simulink library "mech_car_library"  (Simulink 7.1)
libraries: mblibv1 x13, mwlibrary x10, simulink x5
settings Model: Creator=dsampson  LastModifiedBy=batserve

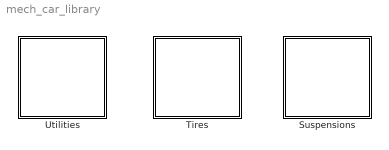
== system mech_car_library ==
  Suspensions : Subsystem
  Tires : Subsystem
  Utilities : Subsystem

== system mech_car_library/Suspensions ==
  Suspension 1 : Subsystem  Orientation=left  mask{r=0.742, d=2, h_u=0.53, k=190e3, b=2025, m_u=706, I_xx_u=0, I_yy_u=440}
      mask prompts: r "Roll centre height [m]:"; d "Track width [m]:"; h_u "Wheel radius [m]:"; k "Suspension stiffness [N/m]:"; b "Suspension damping [N.s/m]:"; m_u "Mass [kg]:"; I_xx_u "Roll inertia [kg.m2]:"; I_yy_u "Yaw inertia [kg.m2]:"
      mask init:
      | I_zz_u = I_xx_u;

== system mech_car_library/Tires ==
  Magic 1 : Subsystem  mask{r_e=0.53, r_f=0.55, m_w=10, F_z=25000, F_x_max=15000, kappa_max=10, F_y_max=15000, alpha_max=10, sigma_k=1.6, kt=1030000}
      mask prompts: r_e "Effective rolling radius [m]:"; r_f "Unloaded radius [m]:"; m_w "Wheel mass [kg]:"; F_z "Rated vertical load [N]:"; F_x_max "Peak longitudinal force at rated load [N]:"; kappa_max "Best slip at rated load [percent]:"; F_y_max "Peak lateral force at rated load [N]:"; alpha_max "Best sideslip at rated load [deg]:"; sigma_k "Relaxation length at rated load [m]:"; kt "Vertical stiffness"

== system mech_car_library/Utilities ==
  Cross Product : Subsystem
      mask Type: Cross Product
      mask Description: Calculate the cross product of two 3x1 vectors.
  Unit Vector : Subsystem
      mask Type: Unit Vector
      mask Description: Normalize a 3x1 vector.

== system mech_car_library/Suspensions/Suspension 1 ==
  Body Spring & Damper : mblibv1/Force  Elements/Body Spring & Damper  Orientation=down  DialogController=MECH.DynMechDlgSource  SystemSampleTime=-1  DialogClass=BodySpringDamper  Spring_k=k  Damper_b=b  Offset_x0=0  PositionUnits=m  VelocityUnits=m/s  ForceUnits=N
  Body Spring & Damper1 : mblibv1/Force  Elements/Body Spring & Damper  Orientation=down  DialogController=MECH.DynMechDlgSource  SystemSampleTime=-1  DialogClass=BodySpringDamper  Spring_k=k  Damper_b=b  Offset_x0=0  PositionUnits=m  VelocityUnits=m/s  ForceUnits=N
  Body1 : mblibv1/Bodies/Body  Orientation=down  DialogController=MECH.DynMechDlgSource  PhysicalDomain=mechanical  SubClassName=Unknown  LeftPortType=workingframe  RightPortType=workingframe  LConnTagsString=CS1|CS2|CS3  RConnTagsString=CS4|CS5  DialogClass=MechanicalBodyBlock  Mass=m_u  MassUnits=kg  InertiaUnits=kg*m^2  Inertia=diag([I_xx_u,I_yy_u,I_zz_u])  Shape=Cylinder  ShapeDims=[1 1]  ShapeUnits=m  ShapeUse=false  Density=1  DensityUnits=kg/m^3  DensityUse=false  GraphicsMode=1  BodyColor=[0.5 0.5 0.5]  GraphicsObj=[]  AttachedToCS=1  CG=Left$CG$[0 0 0]$CS2$CS2$m$[0 0 0]$Euler X-Y-Z$deg$WORLD$false  WorkingFrames=Left$CS1$[0,d/2,0]$CS2$CS2$m$[0 0 0]$Euler X-Y-Z$deg$WORLD$true#Left$CS2$[0,0,0]$ADJOINING$ADJOINING$m$[0 0 0]$Euler X-Y-Z$deg$WORLD$true#Left$CS3$[0,-d/2,0]$CS2$CS2$m$[0 0 0]$Euler X-Y-Z$deg$WORLD$true#Right$CS4$[0,d/2,h_u-r]$CS2$CS2$m$[0 0 0]$Euler X-Y-Z$deg$WORLD$true#Right$CS5$[0,-d/2,h_u-r]$CS2$CS2$m$[0 0 0]$Euler X-Y-Z$deg$WORLD$true  CGPos=[0 0 0]  CGRot=[0 0 0]  CS0Pos=[]  CS0Rot=[]  CS1Pos=[0 0 0]  CS1Rot=[0 0 0]  CS2Pos=[0 0 0]  CS2Rot=[0 0 0]  CS3Pos=[]  CS3Rot=[]  CS4Pos=[]  CS4Rot=[]  CS5Pos=[]  CS5Rot=[]  CS6Pos=[]  CS6Rot=[]  CS7Pos=[]  CS7Rot=[]  CS8Pos=[]  CS8Rot=[]  CS9Pos=[]  CS9Rot=[]  CS10Pos=[]  CS10Rot=[]  CS11Pos=[]  CS11Rot=[]  CS12Pos=[]  CS12Rot=[]  CS13Pos=[]  CS13Rot=[]  CS14Pos=[]  CS14Rot=[]  CS15Pos=[]  CS15Rot=[]  CS16Pos=[]  CS16Rot=[]  CS17Pos=[]  CS17Rot=[]  CS18Pos=[]  CS18Rot=[]  CS19Pos=[]  CS19Rot=[]  CS20Pos=[]  CS20Rot=[]
  Custom Joint : mblibv1/Joints/Custom Joint  Orientation=down  DialogController=MECH.DynMechDlgSource  PhysicalDomain=mechanical  SubClassName=custom_joint  LeftPortType=blob  RightPortType=blob  LConnTagsString=__newl0  RConnTagsString=__newr0  NumSAPorts=0  CutJoint=off  MarkAsCut=off  Primitives=prismatic_revolute  PrimitiveProps=P1$Base$[0 0 1]$prismatic#R1$Base$[1 0 0]$revolute  DialogClass=JointBlock  R1Axis=[1 0 0]  R2Axis=[]  R3Axis=[]  P1Axis=[]  P2Axis=[]  P3Axis=[]  SAxis=[]
  Left Spring : PMIOPort  Orientation=down  Port=1  Side=Left
  Joint : PMIOPort  Orientation=down  Port=2  Side=Left
  Right Spring : PMIOPort  Orientation=down  Port=3  Side=Left
  Left Wheel : PMIOPort  Orientation=up  Port=4  Side=Right
  Right Wheel : PMIOPort  Orientation=up  Port=5  Side=Right
  connections:
  Body Spring & Damper/RConn1 -- Body1/LConn1
  Body Spring & Damper1/RConn1 -- Body1/LConn3
  Custom Joint/RConn1 -- Body1/LConn2
  Left Spring/RConn1 -- Body Spring & Damper/LConn1
  Right Spring/RConn1 -- Body Spring & Damper1/LConn1
  Joint/RConn1 -- Custom Joint/LConn1
  Left Wheel/RConn1 -- Body1/RConn1
  Right Wheel/RConn1 -- Body1/RConn2

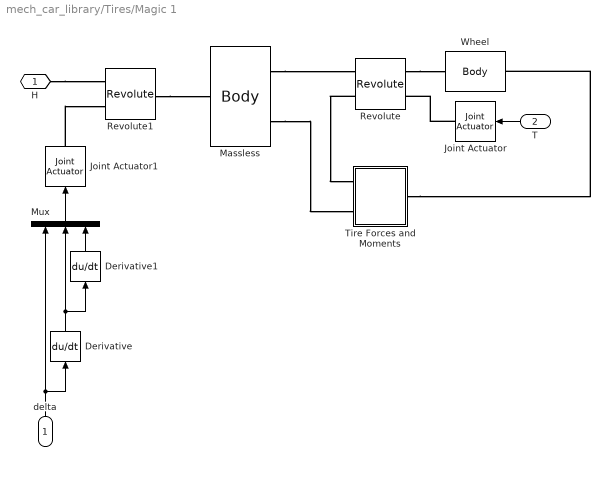
== system mech_car_library/Tires/Magic 1 ==
  delta : Inport  Orientation=up  OutDataType=sfix(16)  OutScaling=2^0
  T : Inport  Orientation=left  Port=2  OutDataType=sfix(16)  OutScaling=2^0
  Derivative : Derivative  Orientation=up
  Derivative1 : Derivative  Orientation=up
  Joint Actuator : mblibv1/Sensors &  Actuators/Joint Actuator  Orientation=left  DialogController=MECH.DynMechDlgSource  SystemSampleTime=-1  PhysicalDomain=Mechanical  PortType=blob  ActuationStyle=Force  AngleUnits=deg  ArcVelocityUnits=deg/s  ArcAccelerationUnits=deg/s^2  CoordPositionUnits=m  VelocityUnits=m/s  AccelerationUnits=m/s^2  ForceUnits=N  TorqueUnits=N-m  ActiveIO=on  Width=1  DialogClass=MechanicalActuatorBlock  Primitive=R1  ReferenceFrame=Absolute (INERTIAL)
  Joint Actuator1 : mblibv1/Sensors &  Actuators/Joint Actuator  Orientation=up  DialogController=MECH.DynMechDlgSource  SystemSampleTime=-1  PhysicalDomain=Mechanical  PortType=blob  ActuationStyle=Motion  AngleUnits=deg  ArcVelocityUnits=deg/s  ArcAccelerationUnits=deg/s^2  CoordPositionUnits=m  VelocityUnits=m/s  AccelerationUnits=m/s^2  ForceUnits=N  TorqueUnits=N-m  ActiveIO=on  Width=3  DialogClass=MechanicalActuatorBlock  Primitive=R1  ReferenceFrame=Absolute (INERTIAL)
  Massless : mblibv1/Bodies/Body  DialogController=MECH.DynMechDlgSource  PhysicalDomain=mechanical  SubClassName=Unknown  LeftPortType=workingframe  RightPortType=workingframe  LConnTagsString=CS1  RConnTagsString=CS2|CS3  DialogClass=MechanicalBodyBlock  Mass=0  MassUnits=kg  InertiaUnits=kg*m^2  Inertia=0*eye(3)  Shape=Cylinder  ShapeDims=[1 1]  ShapeUnits=m  ShapeUse=false  Density=1  DensityUnits=kg/m^3  DensityUse=false  GraphicsMode=1  BodyColor=[0.5 0.5 0.5]  GraphicsObj=[]  AttachedToCS=1  CG=Left$CG$[0 0 0]$CS1$CS1$m$[0 0 0]$Euler X-Y-Z$deg$WORLD$false  WorkingFrames=Left$CS1$[0 0 0]$ADJOINING$ADJOINING$m$[0 0 0]$Euler X-Y-Z$deg$WORLD$true#Right$CS2$[0 0 0]$CG$CG$m$[0 0 0]$Euler X-Y-Z$deg$WORLD$true#Right$CS3$[0 0 0]$CG$CG$m$[0 0 0]$Euler X-Y-Z$deg$WORLD$true  CGPos=[0 0 0]  CGRot=[0 0 0]  CS0Pos=[]  CS0Rot=[]  CS1Pos=[0 0 0]  CS1Rot=[0 0 0]  CS2Pos=[0 0 0]  CS2Rot=[0 0 0]  CS3Pos=[]  CS3Rot=[]  CS4Pos=[]  CS4Rot=[]  CS5Pos=[]  CS5Rot=[]  CS6Pos=[]  CS6Rot=[]  CS7Pos=[]  CS7Rot=[]  CS8Pos=[]  CS8Rot=[]  CS9Pos=[]  CS9Rot=[]  CS10Pos=[]  CS10Rot=[]  CS11Pos=[]  CS11Rot=[]  CS12Pos=[]  CS12Rot=[]  CS13Pos=[]  CS13Rot=[]  CS14Pos=[]  CS14Rot=[]  CS15Pos=[]  CS15Rot=[]  CS16Pos=[]  CS16Rot=[]  CS17Pos=[]  CS17Rot=[]  CS18Pos=[]  CS18Rot=[]  CS19Pos=[]  CS19Rot=[]  CS20Pos=[]  CS20Rot=[]
  Mux : Mux  Orientation=up  Inputs=3
  Revolute : mblibv1/Joints/Revolute  DialogController=MECH.DynMechDlgSource  PhysicalDomain=mechanical  SubClassName=Unknown  LeftPortType=blob  RightPortType=blob  LConnTagsString=__newl0|SA1  RConnTagsString=__newr0|SA1  NumSAPorts=2  CutJoint=off  MarkAsCut=off  Primitives=revolute  PrimitiveProps=R1$Base$[0 1 0]$revolute  DialogClass=JointBlock  R1Axis=[0 0 1]
  Revolute1 : mblibv1/Joints/Revolute  DialogController=MECH.DynMechDlgSource  PhysicalDomain=mechanical  SubClassName=Unknown  LeftPortType=blob  RightPortType=blob  LConnTagsString=__newl0|SA1  RConnTagsString=__newr0  NumSAPorts=1  CutJoint=off  MarkAsCut=off  Primitives=revolute  PrimitiveProps=R1$Base$[0 0 1]$revolute  DialogClass=JointBlock  R1Axis=[0 0 1]
  Tire Forces and Moments : Subsystem
  Wheel : mblibv1/Bodies/Body  DialogController=MECH.DynMechDlgSource  PhysicalDomain=mechanical  SubClassName=Unknown  LeftPortType=workingframe  RightPortType=workingframe  LConnTagsString=CS1  RConnTagsString=CS2  DialogClass=MechanicalBodyBlock  Mass=m_w  MassUnits=kg  InertiaUnits=kg*m^2  Inertia=m_w*r_e^2*diag([0.25,0.5,0.25])  Shape=Cylinder  ShapeDims=[1 1]  ShapeUnits=m  ShapeUse=false  Density=1  DensityUnits=kg/m^3  DensityUse=false  GraphicsMode=1  BodyColor=[0.5 0.5 0.5]  GraphicsObj=[]  AttachedToCS=1  CG=Left$CG$[0 0 0]$CS1$CS1$m$[0 0 0]$Euler X-Y-Z$deg$WORLD$false  WorkingFrames=Left$CS1$[0 0 0]$ADJOINING$ADJOINING$m$[0 0 0]$Euler X-Y-Z$deg$WORLD$true#Right$CS2$[0 0 0]$CG$CG$m$[0 0 0]$Euler X-Y-Z$deg$WORLD$true#Right$CS3$[0 0 r_e]$CG$CG$m$[0 0 0]$Euler X-Y-Z$deg$WORLD$false#Right$CS4$[0 0 -r_e]$CG$CG$m$[0 0 0]$Euler X-Y-Z$deg$WORLD$false  CGPos=[0 0 0]  CGRot=[0 0 0]  CS0Pos=[]  CS0Rot=[]  CS1Pos=[0 0 0]  CS1Rot=[0 0 0]  CS2Pos=[0 0 0]  CS2Rot=[0 0 0]  CS3Pos=[]  CS3Rot=[]  CS4Pos=[]  CS4Rot=[]  CS5Pos=[]  CS5Rot=[]  CS6Pos=[]  CS6Rot=[]  CS7Pos=[]  CS7Rot=[]  CS8Pos=[]  CS8Rot=[]  CS9Pos=[]  CS9Rot=[]  CS10Pos=[]  CS10Rot=[]  CS11Pos=[]  CS11Rot=[]  CS12Pos=[]  CS12Rot=[]  CS13Pos=[]  CS13Rot=[]  CS14Pos=[]  CS14Rot=[]  CS15Pos=[]  CS15Rot=[]  CS16Pos=[]  CS16Rot=[]  CS17Pos=[]  CS17Rot=[]  CS18Pos=[]  CS18Rot=[]  CS19Pos=[]  CS19Rot=[]  CS20Pos=[]  CS20Rot=[]
  H : PMIOPort  Port=1  Side=Left
  wires:
  Derivative1/1 -> Mux/3
  Derivative/1 -> Derivative1/1, Mux/2
  delta/1 -> Derivative/1, Mux/1
  Mux/1 -> Joint Actuator1/1
  T/1 -> Joint Actuator/1
  connections:
  Revolute1/RConn1 -- Massless/LConn1
  Revolute/RConn1 -- Wheel/LConn1
  Massless/RConn1 -- Revolute/LConn1
  Joint Actuator/RConn1 -- Revolute/RConn2
  Tire Forces and Moments/RConn1 -- Wheel/RConn1
  H/RConn1 -- Revolute1/LConn1
  Joint Actuator1/RConn1 -- Revolute1/LConn2
  Revolute/LConn2 -- Tire Forces and Moments/LConn1
  Massless/RConn2 -- Tire Forces and Moments/LConn2

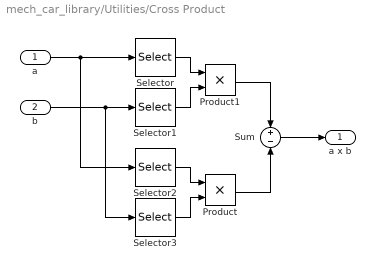
== system mech_car_library/Utilities/Cross Product ==
  a : Inport  PortDimensions=3  OutDataType=sfix(16)  OutScaling=2^0
  b : Inport  Port=2  PortDimensions=3  OutDataType=sfix(16)  OutScaling=2^0
  Product : Product  OutDataType=sfix(16)  OutScaling=2^0  RndMeth=Zero
  Product1 : Product  OutDataType=sfix(16)  OutScaling=2^0  RndMeth=Zero
  Selector : Selector  InputPortWidth=3  IndexOptions=Index vector (dialog)  Indices=[2 3 1]  OutputSizes=1
  Selector1 : Selector  InputPortWidth=3  IndexOptions=Index vector (dialog)  Indices=[3 1 2]  OutputSizes=1
  Selector2 : Selector  InputPortWidth=3  IndexOptions=Index vector (dialog)  Indices=[3 1 2]  OutputSizes=1
  Selector3 : Selector  InputPortWidth=3  IndexOptions=Index vector (dialog)  Indices=[2 3 1]  OutputSizes=1
  Sum : Sum  Inputs=+|-  OutDataType=sfix(16)  OutScaling=2^0
  a x b : Outport  OutDataType=sfix(16)  OutScaling=2^0
  wires:
  Selector2/1 -> Product/1
  Selector3/1 -> Product/2
  Selector/1 -> Product1/1
  Selector1/1 -> Product1/2
  a/1 -> Selector/1, Selector2/1
  b/1 -> Selector1/1, Selector3/1
  Product1/1 -> Sum/1
  Product/1 -> Sum/2
  Sum/1 -> a x b/1

== system mech_car_library/Utilities/Unit Vector ==
  u : Inport  PortDimensions=3  OutDataType=sfix(16)  OutScaling=2^0
  Assertion : Assertion  Enabled=on  AssertionFailFcn=error('Magnitude of input is zero.')
  Normalize l : Fcn  Expr=sqrt(u[1]^2+u[2]^2+u[3]^2)
  Product : Product  Inputs=/*  OutDataType=sfix(16)  OutScaling=2^0  RndMeth=Zero
  u/|u| : Outport  OutDataType=sfix(16)  OutScaling=2^0
  wires:
  u/1 -> Normalize l/1, Product/2
  Normalize l/1 -> Product/1, Assertion/1
  Product/1 -> u/|u|/1

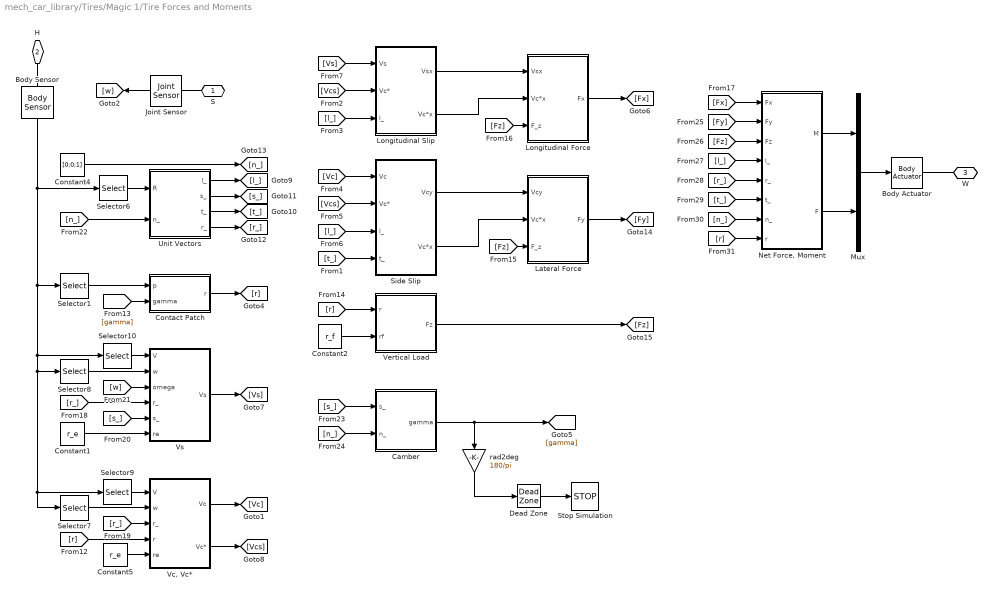
== system mech_car_library/Tires/Magic 1/Tire Forces and Moments ==
  Body Actuator : mblibv1/Sensors &  Actuators/Body Actuator  DialogController=MECH.DynMechDlgSource  SystemSampleTime=-1  PhysicalDomain=Mechanical  PortType=blob  ActuationStyle=Force  AngleUnits=deg  ArcVelocityUnits=deg/s  ArcAccelerationUnits=deg/s^2  CoordPositionUnits=m  VelocityUnits=m/s  AccelerationUnits=m/s^2  ForceUnits=N  TorqueUnits=N-m  ActiveIO=on  Width=6  DialogClass=MechanicalActuatorBlock  ReferenceFrame=Absolute (World)  Angle=off  CoordPosition=on  Force=on  Torque=on
  Body Sensor : mblibv1/Sensors &  Actuators/Body Sensor  Orientation=down  DialogController=MECH.DynMechDlgSource  SystemSampleTime=-1  PhysicalDomain=Mechanical  PortType=blob  Muxed=on  Pose=on  Angle=on  AngleUnits=deg  ArcVelocity=on  ArcVelocityUnits=rad/s  ArcAcceleration=off  ArcAccelerationUnits=rad/s^2  CoordPosition=on  CoordPositionUnits=m  Velocity=on  VelocityUnits=m/s  Acceleration=off  AccelerationUnits=m/s^2  Quaternion=on  QuaternionDT=off  QuaternionDDT=off  QuaternionUnits=off  OutputVector=[ 3 3 3 9 ]  ActiveIO=on  Width=18  DialogClass=MechanicalSensorBlock  ReferenceFrame=Absolute (World)
  Camber : Subsystem
  Constant1 : Constant  Value=r_e  OutDataType=sfix(16)  OutScaling=2^0
  Constant2 : Constant  Value=r_f  OutDataType=sfix(16)  OutScaling=2^0
  Constant4 : Constant  Value=[0;0;1]  OutDataType=sfix(16)  OutScaling=2^0
  Constant5 : Constant  Value=r_e  OutDataType=sfix(16)  OutScaling=2^0
  Contact Patch : Subsystem
  Dead Zone : DeadZone  LowerValue=-70  UpperValue=70  ZeroCross=off  SaturateOnIntegerOverflow=on
  Joint Sensor : mblibv1/Sensors &  Actuators/Joint Sensor  Orientation=left  DialogController=MECH.DynMechDlgSource  SystemSampleTime=-1  PhysicalDomain=Mechanical  PortType=blob  Muxed=on  Pose=off  Angle=off  AngleUnits=deg  ArcVelocity=on  ArcVelocityUnits=rad/s  ArcAcceleration=off  ArcAccelerationUnits=deg/s^2  CoordPosition=on  CoordPositionUnits=m  Velocity=off  VelocityUnits=m/s  Acceleration=off  AccelerationUnits=m/s^2  Quaternion=on  QuaternionDT=off  QuaternionDDT=off  QuaternionUnits=off  OutputVector=[ 1 ]  ActiveIO=on  Width=1  DialogClass=MechanicalSensorBlock  Primitive=R1  Force=off  ForceUnits=N  Torque=off  TorqueUnits=N-m  ReferenceFrame=Absolute (INERTIAL)  ReactionSensedSide=Base  ReactionReferenceFrame=Absolute (World)  ReactionForce=off  ReactionForceUnits=N  ReactionMoment=off  ReactionMomentUnits=N-m
  Lateral Force : Subsystem  mask(Tire Lateral Force){F_z=F_z, F_y_max=F_y_max, alpha_max=alpha_max}
      mask prompts: F_z "Rated vertical load [N]:"; F_y_max "Peak lateral force at rated load [N]:"; alpha_max "Slip at peak force at rated load [degrees]:"
      mask init:
      | % Scaling factors
      | F_z_sf = F_z/3139.2;
      | F_y_sf = F_y_max/3564.1;
      | alpha_sf = alpha_max/9.99;
      | % Magic formula parameters
      | a1 = -24.1;
      | a2 = 1211;
      | a3 = 1178;
      | a4 = 1.82;
      | a5 = 0.208;
      | a6 = 0;
      | a7 = -0.354;
      | a8 = 0.707;
      | % Lookup table parameters
      | alpha_bp = [0:0.1:19.9 20:1:50];
      | F_z_bp = linspace(0,2*max(F_z(:)),101);
      | [alpha_grid, F_z_grid] = meshgrid(alpha_bp, F_z_bp);
      | F_y_grid = tire_Fy(alpha_grid, F_z_grid, a1, a2, a3, a4, a5, a6, a7, a8);
  Longitudinal Force : Subsystem  mask(Tire Longitudinal Force){F_z=F_z, F_x_max=F_x_max, kappa_max=kappa_max, sigma_k=sigma_k}
      mask prompts: F_z "Rated vertical load [N]:"; F_x_max "Peak longitudinal force at rated load [N]:"; kappa_max "Slip at peak force at rated load [percent]:"; sigma_k "Relaxation length at rated load [m]:"
      mask init:
      | % Scaling factors
      | F_z_sf = F_z/3139.2;
      | F_x_sf = F_x_max/3381.3;
      | kappa_sf = kappa_max/10.93;
      | % Magic formula parameters
      | a1 = -21.3;
      | a2 = 1144;
      | a3 = 49.6;
      | a4 = 226;
      | a5 = 0.069;
      | a6 = -0.006;
      | a7 = 0.056;
      | a8 = 0.486;
      | % Small-perturbation coefficients
      | D_x = a1*(F_z/1000)^2 + a2*(F_z/1000);
      | C_x = 1.65;
      | B_x = ((a3*(F_z/1000)^2 + a4*(F_z/1000)) / (C_x*D_x*exp(a5*(F_z/1000))))*100;
      | E_x = a6*(F_z/1000)^2 + a7*(F_z/1000) + a8;
      | C_fk = B_x * C_x * D_x * F_x_sf / kappa_sf;
      | C_fx = C_fk / sigma_k;
      | % Low speed damping coefficients
      | sigma_min = 0.02;
      | k_V_low0 = 770;
      | V_low = 2.5;
      | % Lookup table parameters
      | kappa_bp = [0:0.01:0.99 1:0.5:5];
      | F_z_bp = linspace(0,2*max(F_z(:)),101);
      | [kappa_grid, F_z_grid] = meshgrid(kappa_bp, F_z_bp);
      | F_x_grid = tire_Fx(kappa_grid, F_z_grid, a1, a2, a3, a4, a5, a6, a7, a8);
      | dFx_dFz_grid = tire_dFx_dFz(kappa_grid, F_z_grid, a1, a2, a3, a4, a5, a6, a7, a8);
      | dFx_dkappa_grid = tire_dFx_dkappa(kappa_grid, F_z_grid, a1, a2, a3, a4, a5, a6, a7, a8);
  Longitudinal Slip : Subsystem
  Mux : Mux  Inputs=2
  "Net Force, Moment" : Subsystem
  Selector1 : Selector  InputPortWidth=18  IndexOptions=Index vector (dialog)  Indices=1:3  OutputSizes=1
  Selector10 : Selector  InputPortWidth=18  IndexOptions=Index vector (dialog)  Indices=4:6  OutputSizes=1
  Selector6 : Selector  InputPortWidth=18  IndexOptions=Index vector (dialog)  Indices=10:18  OutputSizes=1
  Selector7 : Selector  InputPortWidth=18  IndexOptions=Index vector (dialog)  Indices=7:9  OutputSizes=1
  Selector8 : Selector  InputPortWidth=18  IndexOptions=Index vector (dialog)  Indices=7:9  OutputSizes=1
  Selector9 : Selector  InputPortWidth=18  IndexOptions=Index vector (dialog)  Indices=4:6  OutputSizes=1
  Side Slip : Subsystem
  Stop Simulation : Stop
  Unit Vectors : Subsystem
  "Vc, Vc*" : Subsystem
  Vertical Load : Subsystem
  Vs : Subsystem
  rad2deg : Gain  Orientation=down  Gain=180/pi  ParameterDataType=sfix(16)  ParameterScaling=2^0  OutDataType=sfix(16)  OutScaling=2^0
  S : PMIOPort  Orientation=left  Port=1  Side=Left
  H : PMIOPort  Orientation=down  Port=2  Side=Left
  W : PMIOPort  Orientation=left  Port=3  Side=Right
  wires:
  Lateral Force/1(Fy) -> [Fy]
  rad2deg/1 -> Dead Zone/1
  Longitudinal Slip/2(Vc*x) -> Longitudinal Force/2(Vc*x)
  Side Slip/2(Vc*x) -> Lateral Force/2(Vc*x)
  Side Slip/1(Vcy) -> Lateral Force/1(Vcy)
  [Vcs] -> Side Slip/2(Vc*)
  [Vc] -> Side Slip/1(Vc)
  [t_] -> Side Slip/4(t_)
  [l_] -> Side Slip/3(l_)
  [l_] -> Longitudinal Slip/3(l_)
  [Vcs] -> Longitudinal Slip/2(Vc*)
  [Vs] -> Longitudinal Slip/1(Vs)
  [r] -> "Vc, Vc*"/4(r)
  "Vc, Vc*"/2(Vc*) -> [Vcs]
  "Vc, Vc*"/1(Vc) -> [Vc]
  Vs/1(Vs) -> [Vs]
  Constant5/1 -> "Vc, Vc*"/5(re)
  [s_] -> Vs/5(s_)
  [r_] -> "Vc, Vc*"/3(r_)
  [r_] -> Vs/4(r_)
  [w] -> Vs/3(omega)
  Selector7/1 -> "Vc, Vc*"/2(w)
  Selector9/1 -> "Vc, Vc*"/1(V)
  Constant1/1 -> Vs/6(re)
  Selector8/1 -> Vs/2(w)
  Selector10/1 -> Vs/1(V)
  [gamma] -> Contact Patch/2(gamma)
  Contact Patch/1(r) -> [r]
  Selector1/1 -> Contact Patch/1(p)
  [n_] -> Unit Vectors/2(n_)
  Constant4/1 -> [n_]
  Unit Vectors/3(t_) -> [t_]
  Unit Vectors/4(r_) -> [r_]
  Unit Vectors/2(s_) -> [s_]
  Unit Vectors/1(l_) -> [l_]
  Selector6/1 -> Unit Vectors/1(R)
  "Net Force, Moment"/2(F) -> Mux/2
  "Net Force, Moment"/1(M) -> Mux/1
  Vertical Load/1(Fz) -> [Fz]
  [r] -> "Net Force, Moment"/8(r)
  [n_] -> "Net Force, Moment"/7(n_)
  [t_] -> "Net Force, Moment"/6(t_)
  [r_] -> "Net Force, Moment"/5(r_)
  [l_] -> "Net Force, Moment"/4(l_)
  [Fz] -> "Net Force, Moment"/3(Fz)
  [Fy] -> "Net Force, Moment"/2(Fy)
  [Fx] -> "Net Force, Moment"/1(Fx)
  [Fz] -> Longitudinal Force/3(F_z)
  [Fz] -> Lateral Force/3(F_z)
  Constant2/1 -> Vertical Load/2(rf)
  [r] -> Vertical Load/1(r)
  Longitudinal Force/1(Fx) -> [Fx]
  Longitudinal Slip/1(Vsx) -> Longitudinal Force/1(Vsx)
  Camber/1(gamma) -> rad2deg/1, [gamma]
  [n_] -> Camber/2(n_)
  [s_] -> Camber/1(s_)
  Joint Sensor/1 -> [w]
  Body Sensor/1 -> Selector7/1, Selector9/1, Selector8/1, Selector10/1, Selector1/1, Selector6/1
  Mux/1 -> Body Actuator/1
  Dead Zone/1 -> Stop Simulation/1
  connections:
  S/RConn1 -- Joint Sensor/LConn1
  H/RConn1 -- Body Sensor/LConn1
  Body Actuator/RConn1 -- W/RConn1

== system mech_car_library/Tires/Magic 1/Tire Forces and Moments/Camber ==
  s_ : Inport  OutDataType=sfix(16)  OutScaling=2^0
  n_ : Inport  Port=2  OutDataType=sfix(16)  OutScaling=2^0
  Dot Product1 : simulink/Math Operations/Dot Product  InputSameDT=on  OutDataType=sfix(16)  OutScaling=2^-10  DoSatur=off
  Trigonometric Function : Trigonometry  Operator=asin
  gamma : Outport  OutDataType=sfix(16)  OutScaling=2^0
  wires:
  n_/1 -> Dot Product1/2
  s_/1 -> Dot Product1/1
  Dot Product1/1 -> Trigonometric Function/1
  Trigonometric Function/1 -> gamma/1

== system mech_car_library/Tires/Magic 1/Tire Forces and Moments/Contact Patch ==
  p : Inport  OutDataType=sfix(16)  OutScaling=2^0
  gamma : Inport  Port=2  OutDataType=sfix(16)  OutScaling=2^0
  Abs : Abs
  Product2 : Product  Inputs=*/  OutDataType=sfix(16)  OutScaling=2^0  RndMeth=Zero
  Selector : Selector  InputPortWidth=3  IndexOptions=Index vector (dialog)  Indices=3  OutputSizes=1
  Trigonometric Function : Trigonometry  Operator=cos
  r : Outport  OutDataType=sfix(16)  OutScaling=2^0
  wires:
  Abs/1 -> r/1
  Product2/1 -> Abs/1
  Trigonometric Function/1 -> Product2/2
  gamma/1 -> Trigonometric Function/1
  Selector/1 -> Product2/1
  p/1 -> Selector/1

== system mech_car_library/Tires/Magic 1/Tire Forces and Moments/Lateral Force ==
  Vcy : Inport  OutDataType=sfix(16)  OutScaling=2^0
  Vc*x : Inport  Port=2  OutDataType=sfix(16)  OutScaling=2^0
  F_z : Inport  Port=3  OutDataType=sfix(16)  OutScaling=2^0
  Slip : Subsystem
  Tire force : Subsystem
  Fy : Outport  OutDataType=sfix(16)  OutScaling=2^0
  wires:
  Vc*x/1 -> Slip/2(Vc*x)
  Vcy/1 -> Slip/1(Vcy)
  Slip/1(alpha) -> Tire force/2(alpha)
  Tire force/1(F_y) -> Fy/1
  F_z/1 -> Tire force/1(F_z)

== system mech_car_library/Tires/Magic 1/Tire Forces and Moments/Longitudinal Force ==
  Vsx : Inport  OutDataType=sfix(16)  OutScaling=2^0
  Vc*x : Inport  Port=2  OutDataType=sfix(16)  OutScaling=2^0
  F_z : Inport  Port=3  OutDataType=sfix(16)  OutScaling=2^0
  Tire force : Subsystem
  Transient slip : Subsystem
  Fx : Outport  OutDataType=sfix(16)  OutScaling=2^0
  wires:
  Vsx/1 -> Transient slip/3(V_sx)
  Vc*x/1 -> Transient slip/2(V_x)
  Transient slip/1(kappa) -> Tire force/2(kappa)
  Tire force/1(F_x) -> Fx/1
  F_z/1 -> Transient slip/1(F_z), Tire force/1(F_z)

== system mech_car_library/Tires/Magic 1/Tire Forces and Moments/Longitudinal Slip ==
  Vs : Inport  OutDataType=sfix(16)  OutScaling=2^0
  Vc* : Inport  Port=2  OutDataType=sfix(16)  OutScaling=2^0
  l_ : Inport  Port=3  OutDataType=sfix(16)  OutScaling=2^0
  Dot Product : simulink/Math Operations/Dot Product  InputSameDT=on  OutDataType=sfix(16)  OutScaling=2^-10  DoSatur=off
  Dot Product1 : simulink/Math Operations/Dot Product  InputSameDT=on  OutDataType=sfix(16)  OutScaling=2^-10  DoSatur=off
  Vsx : Outport  OutDataType=sfix(16)  OutScaling=2^0
  Vc*x : Outport  Port=2  OutDataType=sfix(16)  OutScaling=2^0
  wires:
  Dot Product1/1 -> Vc*x/1
  Dot Product/1 -> Vsx/1
  Vc*/1 -> Dot Product1/2
  l_/1 -> Dot Product1/1, Dot Product/2
  Vs/1 -> Dot Product/1

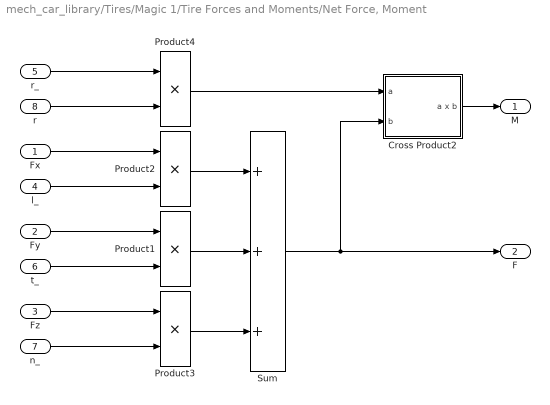
== system mech_car_library/Tires/Magic 1/Tire Forces and Moments/Net Force, Moment ==
  Fx : Inport  OutDataType=sfix(16)  OutScaling=2^0
  Fy : Inport  Port=2  OutDataType=sfix(16)  OutScaling=2^0
  Fz : Inport  Port=3  OutDataType=sfix(16)  OutScaling=2^0
  l_ : Inport  Port=4  OutDataType=sfix(16)  OutScaling=2^0
  r_ : Inport  Port=5  OutDataType=sfix(16)  OutScaling=2^0
  t_ : Inport  Port=6  OutDataType=sfix(16)  OutScaling=2^0
  n_ : Inport  Port=7  OutDataType=sfix(16)  OutScaling=2^0
  r : Inport  Port=8  OutDataType=sfix(16)  OutScaling=2^0
  Cross Product2 : Subsystem
  Product{1..4} (4 alike) : Product  OutDataType=sfix(16)  OutScaling=2^0  RndMeth=Zero
  Sum : Sum  Inputs=+++  OutDataType=sfix(16)  OutScaling=2^0
  M : Outport  OutDataType=sfix(16)  OutScaling=2^0
  F : Outport  Port=2  OutDataType=sfix(16)  OutScaling=2^0
  wires:
  Cross Product2/1(a x b) -> M/1
  Product4/1 -> Cross Product2/1(a)
  Sum/1 -> F/1, Cross Product2/2(b)
  Product3/1 -> Sum/3
  Product1/1 -> Sum/2
  Product2/1 -> Sum/1
  r/1 -> Product4/2
  r_/1 -> Product4/1
  n_/1 -> Product3/2
  Fz/1 -> Product3/1
  t_/1 -> Product1/2
  Fy/1 -> Product1/1
  l_/1 -> Product2/2
  Fx/1 -> Product2/1

== system mech_car_library/Tires/Magic 1/Tire Forces and Moments/Side Slip ==
  Vc : Inport  OutDataType=sfix(16)  OutScaling=2^0
  Vc* : Inport  Port=2  OutDataType=sfix(16)  OutScaling=2^0
  l_ : Inport  Port=3  OutDataType=sfix(16)  OutScaling=2^0
  t_ : Inport  Port=4  OutDataType=sfix(16)  OutScaling=2^0
  Dot Product : simulink/Math Operations/Dot Product  InputSameDT=on  OutDataType=sfix(16)  OutScaling=2^-10  DoSatur=off
  Dot Product1 : simulink/Math Operations/Dot Product  InputSameDT=on  OutDataType=sfix(16)  OutScaling=2^-10  DoSatur=off
  Vcy : Outport  OutDataType=sfix(16)  OutScaling=2^0
  Vc*x : Outport  Port=2  OutDataType=sfix(16)  OutScaling=2^0
  wires:
  Dot Product/1 -> Vc*x/1
  Dot Product1/1 -> Vcy/1
  t_/1 -> Dot Product1/2
  Vc/1 -> Dot Product1/1
  Vc*/1 -> Dot Product/1
  l_/1 -> Dot Product/2

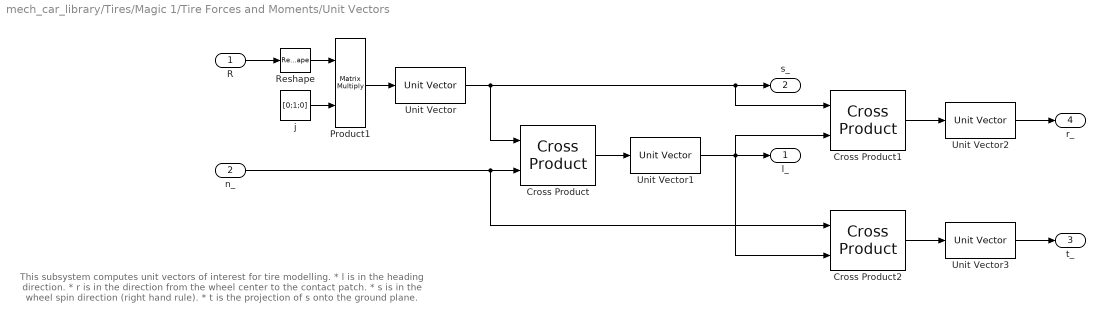
== system mech_car_library/Tires/Magic 1/Tire Forces and Moments/Unit Vectors ==
  note: This subsystem computes unit vectors of interest for tire modelling.
      | * l is in the heading direction.
      | * r is in the direction from the wheel center to the contact patch.
      | * s is in the wheel spin direction (right hand rule).
      | * t is the projection of s onto the ground plane.
  R : Inport  OutDataType=sfix(16)  OutScaling=2^0
  n_ : Inport  Port=2  OutDataType=sfix(16)  OutScaling=2^0
  Cross Product : mwlibrary/Utilities/Cross Product
  Cross Product1 : mwlibrary/Utilities/Cross Product
  Cross Product2 : mwlibrary/Utilities/Cross Product
  Product1 : Product  Multiplication=Matrix(*)  OutDataType=sfix(16)  OutScaling=2^0  RndMeth=Zero
  Reshape : Reshape  OutputDimensionality=Customize  OutputDimensions=[3,3]
  Unit Vector{,1..3} (4 alike) : mwlibrary/Utilities/Unit Vector
  j : Constant  Value=[0;1;0]  OutDataType=sfix(16)  OutScaling=2^0
  l_ : Outport  OutDataType=sfix(16)  OutScaling=2^0
  s_ : Outport  Port=2  OutDataType=sfix(16)  OutScaling=2^0
  t_ : Outport  Port=3  OutDataType=sfix(16)  OutScaling=2^0
  r_ : Outport  Port=4  OutDataType=sfix(16)  OutScaling=2^0
  wires:
  Unit Vector1/1 -> Cross Product2/2, Cross Product1/2, l_/1
  Cross Product/1 -> Unit Vector1/1
  n_/1 -> Cross Product2/1, Cross Product/2
  Unit Vector2/1 -> r_/1
  Cross Product1/1 -> Unit Vector2/1
  Unit Vector3/1 -> t_/1
  Cross Product2/1 -> Unit Vector3/1
  Unit Vector/1 -> Cross Product/1, Cross Product1/1, s_/1
  Product1/1 -> Unit Vector/1
  Reshape/1 -> Product1/1
  R/1 -> Reshape/1
  j/1 -> Product1/2

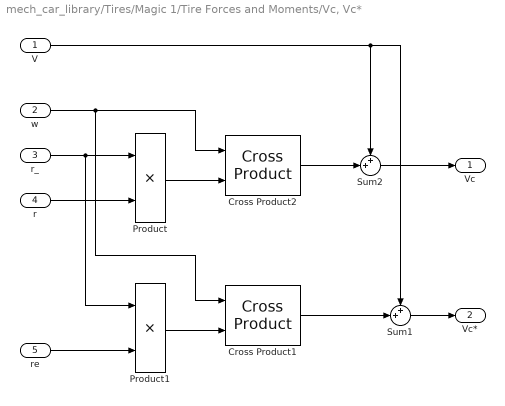
== system mech_car_library/Tires/Magic 1/Tire Forces and Moments/Vc, Vc* ==
  V : Inport  OutDataType=sfix(16)  OutScaling=2^0
  w : Inport  Port=2  OutDataType=sfix(16)  OutScaling=2^0
  r_ : Inport  Port=3  OutDataType=sfix(16)  OutScaling=2^0
  r : Inport  Port=4  OutDataType=sfix(16)  OutScaling=2^0
  re : Inport  Port=5  OutDataType=sfix(16)  OutScaling=2^0
  Cross Product1 : mwlibrary/Utilities/Cross Product
  Cross Product2 : mwlibrary/Utilities/Cross Product
  Product : Product  OutDataType=sfix(16)  OutScaling=2^0  RndMeth=Zero
  Product1 : Product  OutDataType=sfix(16)  OutScaling=2^0  RndMeth=Zero
  Sum1 : Sum  Inputs=++|  OutDataType=sfix(16)  OutScaling=2^0
  Sum2 : Sum  Inputs=++|  OutDataType=sfix(16)  OutScaling=2^0
  Vc : Outport  OutDataType=sfix(16)  OutScaling=2^0
  Vc* : Outport  Port=2  OutDataType=sfix(16)  OutScaling=2^0
  wires:
  Cross Product1/1 -> Sum1/2
  Cross Product2/1 -> Sum2/2
  Sum1/1 -> Vc*/1
  Sum2/1 -> Vc/1
  re/1 -> Product1/2
  Product1/1 -> Cross Product1/2
  V/1 -> Sum1/1, Sum2/1
  Product/1 -> Cross Product2/2
  r/1 -> Product/2
  r_/1 -> Product1/1, Product/1
  w/1 -> Cross Product1/1, Cross Product2/1

== system mech_car_library/Tires/Magic 1/Tire Forces and Moments/Vertical Load ==
  r : Inport  OutDataType=sfix(16)  OutScaling=2^0
  rf : Inport  Port=2  OutDataType=sfix(16)  OutScaling=2^0
  Gain : Gain  Gain=kt  ParameterDataType=sfix(16)  ParameterScaling=2^0  OutDataType=sfix(16)  OutScaling=2^0
  Saturation : Saturate  UpperLimit=Inf  LowerLimit=0  ZeroCross=off
  Sum : Sum  Inputs=|-+  OutDataType=sfix(16)  OutScaling=2^0
  Fz : Outport  OutDataType=sfix(16)  OutScaling=2^0
  wires:
  Saturation/1 -> Fz/1
  Gain/1 -> Saturation/1
  Sum/1 -> Gain/1
  rf/1 -> Sum/2
  r/1 -> Sum/1

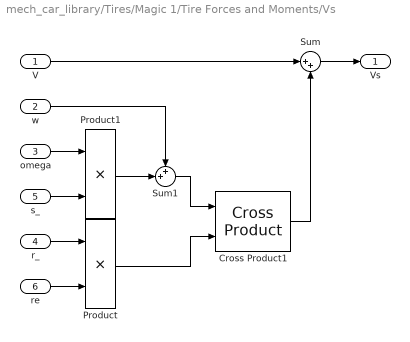
== system mech_car_library/Tires/Magic 1/Tire Forces and Moments/Vs ==
  V : Inport  OutDataType=sfix(16)  OutScaling=2^0
  w : Inport  Port=2  OutDataType=sfix(16)  OutScaling=2^0
  omega : Inport  Port=3  OutDataType=sfix(16)  OutScaling=2^0
  r_ : Inport  Port=4  OutDataType=sfix(16)  OutScaling=2^0
  s_ : Inport  Port=5  OutDataType=sfix(16)  OutScaling=2^0
  re : Inport  Port=6  OutDataType=sfix(16)  OutScaling=2^0
  Cross Product1 : mwlibrary/Utilities/Cross Product
  Product : Product  OutDataType=sfix(16)  OutScaling=2^0  RndMeth=Zero
  Product1 : Product  OutDataType=sfix(16)  OutScaling=2^0  RndMeth=Zero
  Sum : Sum  Inputs=|++  OutDataType=sfix(16)  OutScaling=2^0
  Sum1 : Sum  Inputs=++|  OutDataType=sfix(16)  OutScaling=2^0
  Vs : Outport  OutDataType=sfix(16)  OutScaling=2^0
  wires:
  r_/1 -> Product/1
  re/1 -> Product/2
  Product/1 -> Cross Product1/2
  V/1 -> Sum/1
  Cross Product1/1 -> Sum/2
  Sum/1 -> Vs/1
  omega/1 -> Product1/1
  s_/1 -> Product1/2
  w/1 -> Sum1/1
  Product1/1 -> Sum1/2
  Sum1/1 -> Cross Product1/1

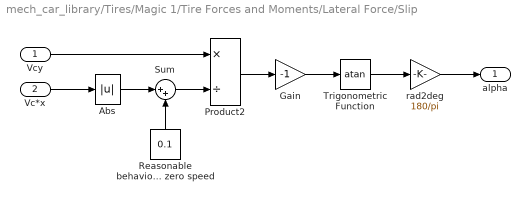
== system mech_car_library/Tires/Magic 1/Tire Forces and Moments/Lateral Force/Slip ==
  Vcy : Inport  OutDataType=sfix(16)  OutScaling=2^0
  Vc*x : Inport  Port=2  OutDataType=sfix(16)  OutScaling=2^0
  Abs : Abs  ZeroCross=off
  Gain : Gain  Gain=-1  ParameterDataType=sfix(16)  ParameterScaling=2^0  OutDataType=sfix(16)  OutScaling=2^0
  Product2 : Product  Inputs=*/  OutDataType=sfix(16)  OutScaling=2^0  RndMeth=Zero
  Reasonable behaviour around zero speed : Constant  Orientation=up  Value=0.1  OutDataType=sfix(16)  OutScaling=2^0
  Sum : Sum  Inputs=|++  OutDataType=sfix(16)  OutScaling=2^0
  Trigonometric Function : Trigonometry  Operator=atan
  rad2deg : Gain  Gain=180/pi  ParameterDataType=sfix(16)  ParameterScaling=2^0  OutDataType=sfix(16)  OutScaling=2^0
  alpha : Outport  OutDataType=sfix(16)  OutScaling=2^0
  wires:
  Vc*x/1 -> Abs/1
  Abs/1 -> Sum/1
  Reasonable behaviour around zero speed/1 -> Sum/2
  rad2deg/1 -> alpha/1
  Vcy/1 -> Product2/1
  Trigonometric Function/1 -> rad2deg/1
  Product2/1 -> Gain/1
  Gain/1 -> Trigonometric Function/1
  Sum/1 -> Product2/2

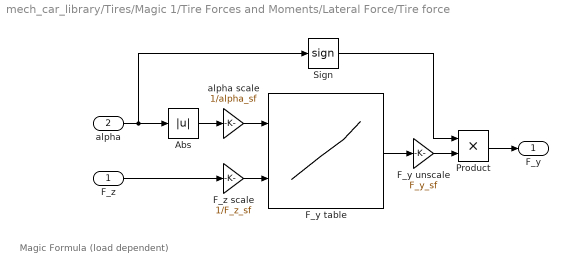
== system mech_car_library/Tires/Magic 1/Tire Forces and Moments/Lateral Force/Tire force ==
  note: Magic Formula (load dependent)
  F_z : Inport  OutDataType=sfix(16)  OutScaling=2^0
  alpha : Inport  Port=2  OutDataType=sfix(16)  OutScaling=2^0
  Abs : Abs  ZeroCross=off
  F_y table : Lookup2D  RowIndex=alpha_bp  ColumnIndex=F_z_bp  Table=F_y_grid'  LookUpMeth=Interpolation-Use End Values  OutDataType=sfix(16)  OutScaling=2^0
  F_y unscale : Gain  Gain=F_y_sf  ParameterDataType=sfix(16)  ParameterScaling=2^0  OutDataType=sfix(16)  OutScaling=2^0
  F_z scale : Gain  Gain=1/F_z_sf  ParameterDataType=sfix(16)  ParameterScaling=2^0  OutDataType=sfix(16)  OutScaling=2^0
  Product : Product  OutDataType=sfix(16)  OutScaling=2^0  RndMeth=Zero
  Sign : Signum  ZeroCross=off
  alpha scale : Gain  Gain=1/alpha_sf  ParameterDataType=sfix(16)  ParameterScaling=2^0  OutDataType=sfix(16)  OutScaling=2^0
  F_y : Outport  OutDataType=sfix(16)  OutScaling=2^0
  wires:
  F_z/1 -> F_z scale/1
  alpha/1 -> Abs/1, Sign/1
  alpha scale/1 -> F_y table/1
  F_z scale/1 -> F_y table/2
  F_y table/1 -> F_y unscale/1
  Abs/1 -> alpha scale/1
  F_y unscale/1 -> Product/2
  Product/1 -> F_y/1
  Sign/1 -> Product/1

== system mech_car_library/Tires/Magic 1/Tire Forces and Moments/Longitudinal Force/Tire force ==
  note: Magic Formula (load dependent)
  F_z : Inport  OutDataType=sfix(16)  OutScaling=2^0
  kappa : Inport  Port=2  OutDataType=sfix(16)  OutScaling=2^0
  Abs : Abs  ZeroCross=off
  F_x table : Lookup2D  RowIndex=kappa_bp  ColumnIndex=F_z_bp  Table=F_x_grid'  LookUpMeth=Interpolation-Use End Values  OutDataType=sfix(16)  OutScaling=2^0
  F_x unscale : Gain  Gain=F_x_sf  ParameterDataType=sfix(16)  ParameterScaling=2^0  OutDataType=sfix(16)  OutScaling=2^0
  F_z scale : Gain  Gain=1/F_z_sf  ParameterDataType=sfix(16)  ParameterScaling=2^0  OutDataType=sfix(16)  OutScaling=2^0
  Product : Product  OutDataType=sfix(16)  OutScaling=2^0  RndMeth=Zero
  Sign : Signum  ZeroCross=off
  kappa scale : Gain  Gain=1/kappa_sf  ParameterDataType=sfix(16)  ParameterScaling=2^0  OutDataType=sfix(16)  OutScaling=2^0
  F_x : Outport  OutDataType=sfix(16)  OutScaling=2^0
  wires:
  F_z/1 -> F_z scale/1
  kappa/1 -> Abs/1, Sign/1
  kappa scale/1 -> F_x table/1
  F_z scale/1 -> F_x table/2
  F_x table/1 -> F_x unscale/1
  Abs/1 -> kappa scale/1
  F_x unscale/1 -> Product/2
  Product/1 -> F_x/1
  Sign/1 -> Product/1

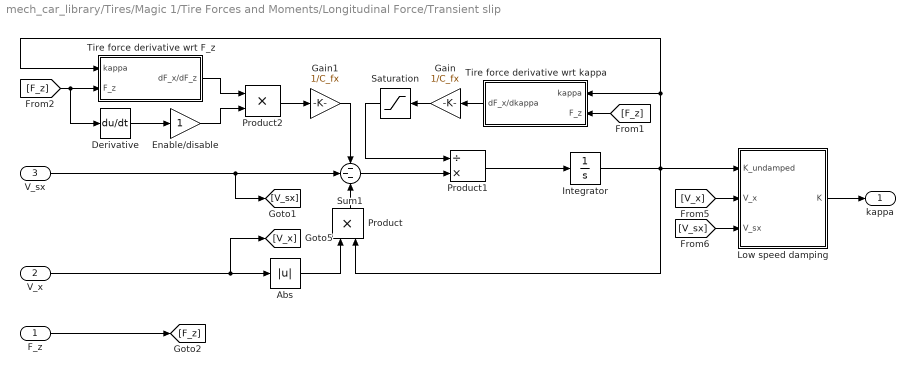
== system mech_car_library/Tires/Magic 1/Tire Forces and Moments/Longitudinal Force/Transient slip ==
  F_z : Inport  OutDataType=sfix(16)  OutScaling=2^0
  V_x : Inport  Port=2  OutDataType=sfix(16)  OutScaling=2^0
  V_sx : Inport  Port=3  OutDataType=sfix(16)  OutScaling=2^0
  Abs : Abs  ZeroCross=off
  Derivative : Derivative
  Enable/disable : Gain  ParameterDataType=sfix(16)  ParameterScaling=2^0  OutDataType=sfix(16)  OutScaling=2^0  SaturateOnIntegerOverflow=on  OutDataTypeStr=Inherit: Same as input  ParamDataTypeStr=Inherit: Same as input
  Gain : Gain  Orientation=left  Gain=1/C_fx  ParameterDataType=sfix(16)  ParameterScaling=2^0  OutDataType=sfix(16)  OutScaling=2^0  SaturateOnIntegerOverflow=on  OutDataTypeStr=Inherit: Same as input  ParamDataTypeStr=Inherit: Same as input
  Gain1 : Gain  Gain=1/C_fx  ParameterDataType=sfix(16)  ParameterScaling=2^0  OutDataType=sfix(16)  OutScaling=2^0  SaturateOnIntegerOverflow=on  OutDataTypeStr=Inherit: Same as input  ParamDataTypeStr=Inherit: Same as input
  Integrator : Integrator  ZeroCross=off
  Low speed damping : Subsystem
  Product : Product  Orientation=up  OutDataType=sfix(16)  OutScaling=2^0  RndMeth=Zero
  Product1 : Product  Inputs=/*  OutDataType=sfix(16)  OutScaling=2^0  RndMeth=Zero
  Product2 : Product  OutDataType=sfix(16)  OutScaling=2^0  RndMeth=Zero
  Saturation : Saturate  Orientation=left  UpperLimit=Inf  LowerLimit=sigma_min  ZeroCross=off
  Sum1 : Sum  Inputs=---  OutDataType=sfix(16)  OutScaling=2^0
  Tire force derivative wrt F_z : Subsystem
  Tire force derivative wrt kappa : Subsystem  Orientation=left
  kappa : Outport  OutDataType=sfix(16)  OutScaling=2^0
  wires:
  V_x/1 -> Abs/1, [V_x]
  V_sx/1 -> [V_sx], Sum1/2
  Abs/1 -> Product/1
  Integrator/1 -> Low speed damping/1(K_undamped), Product/2, Tire force derivative wrt F_z/1(kappa), Tire force derivative wrt kappa/1(kappa)
  Sum1/1 -> Product1/2
  Product1/1 -> Integrator/1
  Gain/1 -> Saturation/1
  Low speed damping/1(K) -> kappa/1
  [V_sx] -> Low speed damping/3(V_sx)
  [V_x] -> Low speed damping/2(V_x)
  Saturation/1 -> Product1/1
  Tire force derivative wrt F_z/1(dF_x/dF_z) -> Product2/1
  Derivative/1 -> Enable/disable/1
  Product/1 -> Sum1/3
  Product2/1 -> Gain1/1
  Gain1/1 -> Sum1/1
  F_z/1 -> [F_z]
  [F_z] -> Derivative/1, Tire force derivative wrt F_z/2(F_z)
  Enable/disable/1 -> Product2/2
  Tire force derivative wrt kappa/1(dF_x/dkappa) -> Gain/1
  [F_z] -> Tire force derivative wrt kappa/2(F_z)

== system mech_car_library/Tires/Magic 1/Tire Forces and Moments/Net Force, Moment/Cross Product2 ==
  a : Inport  OutDataType=sfix(16)  OutScaling=2^0
  b : Inport  Port=2  OutDataType=sfix(16)  OutScaling=2^0
  Product : Product  OutDataType=sfix(16)  OutScaling=2^0  RndMeth=Zero
  Product1 : Product  OutDataType=sfix(16)  OutScaling=2^0  RndMeth=Zero
  Selector : Selector  InputPortWidth=3  IndexOptions=Index vector (dialog)  Indices=[2 3 1]  OutputSizes=1
  Selector1 : Selector  InputPortWidth=3  IndexOptions=Index vector (dialog)  Indices=[3 1 2]  OutputSizes=1
  Selector2 : Selector  InputPortWidth=3  IndexOptions=Index vector (dialog)  Indices=[3 1 2]  OutputSizes=1
  Selector3 : Selector  InputPortWidth=3  IndexOptions=Index vector (dialog)  Indices=[2 3 1]  OutputSizes=1
  Sum : Sum  Inputs=+|-  OutDataType=sfix(16)  OutScaling=2^0
  a x b : Outport  OutDataType=sfix(16)  OutScaling=2^0
  wires:
  Selector2/1 -> Product/1
  Selector3/1 -> Product/2
  Selector/1 -> Product1/1
  Selector1/1 -> Product1/2
  a/1 -> Selector/1, Selector2/1
  b/1 -> Selector1/1, Selector3/1
  Product1/1 -> Sum/1
  Product/1 -> Sum/2
  Sum/1 -> a x b/1

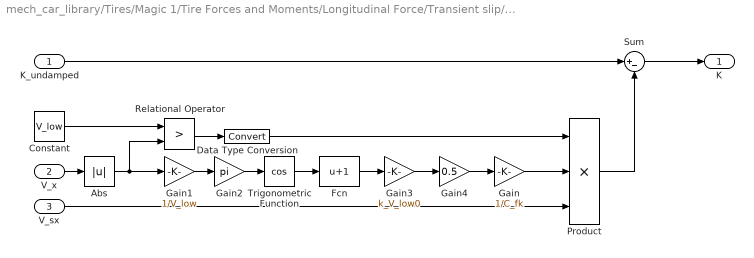
== system mech_car_library/Tires/Magic 1/Tire Forces and Moments/Longitudinal Force/Transient slip/Low speed damping ==
  K_undamped : Inport  OutDataType=sfix(16)  OutScaling=2^0
  V_x : Inport  Port=2  OutDataType=sfix(16)  OutScaling=2^0
  V_sx : Inport  Port=3  OutDataType=sfix(16)  OutScaling=2^0
  Abs : Abs  ZeroCross=off
  Constant : Constant  Value=V_low  OutDataType=sfix(16)  OutScaling=2^0
  Data Type Conversion : DataTypeConversion  OutDataType=sfix(16)  OutScaling=2^0  RndMeth=Zero
  Fcn : Fcn  Expr=u+1
  Gain : Gain  Gain=1/C_fk  ParameterDataType=sfix(16)  ParameterScaling=2^0  OutDataType=sfix(16)  OutScaling=2^0
  Gain1 : Gain  Gain=1/V_low  ParameterDataType=sfix(16)  ParameterScaling=2^0  OutDataType=sfix(16)  OutScaling=2^0
  Gain2 : Gain  Gain=pi  ParameterDataType=sfix(16)  ParameterScaling=2^0  OutDataType=sfix(16)  OutScaling=2^0
  Gain3 : Gain  Gain=k_V_low0  ParameterDataType=sfix(16)  ParameterScaling=2^0  OutDataType=sfix(16)  OutScaling=2^0
  Gain4 : Gain  Gain=0.5  ParameterDataType=sfix(16)  ParameterScaling=2^0  OutDataType=sfix(16)  OutScaling=2^0
  Product : Product  Inputs=3  OutDataType=sfix(16)  OutScaling=2^0  RndMeth=Zero
  Relational Operator : RelationalOperator  Operator=>  LogicOutDataTypeMode=boolean  OutDataTypeStr=boolean  ZeroCross=off
  Sum : Sum  Inputs=|+-  OutDataType=sfix(16)  OutScaling=2^0
  Trigonometric Function : Trigonometry  Operator=cos
  K : Outport  OutDataType=sfix(16)  OutScaling=2^0
  wires:
  V_sx/1 -> Product/3
  Gain/1 -> Product/2
  Data Type Conversion/1 -> Product/1
  Relational Operator/1 -> Data Type Conversion/1
  Constant/1 -> Relational Operator/1
  Gain4/1 -> Gain/1
  Abs/1 -> Relational Operator/2, Gain1/1
  V_x/1 -> Abs/1
  Gain3/1 -> Gain4/1
  Fcn/1 -> Gain3/1
  Trigonometric Function/1 -> Fcn/1
  Gain2/1 -> Trigonometric Function/1
  Gain1/1 -> Gain2/1
  Product/1 -> Sum/2
  Sum/1 -> K/1
  K_undamped/1 -> Sum/1

== system mech_car_library/Tires/Magic 1/Tire Forces and Moments/Longitudinal Force/Transient slip/Tire force derivative wrt F_z ==
  note: Numerical differentiation of the Magic Formula
  kappa : Inport  OutDataType=sfix(16)  OutScaling=2^0
  F_z : Inport  Port=2  OutDataType=sfix(16)  OutScaling=2^0
  Abs : Abs  ZeroCross=off
  F_x unscale : Gain  Gain=F_x_sf  ParameterDataType=sfix(16)  ParameterScaling=2^0  OutDataType=sfix(16)  OutScaling=2^0
  F_z scale : Gain  Gain=1/F_z_sf  ParameterDataType=sfix(16)  ParameterScaling=2^0  OutDataType=sfix(16)  OutScaling=2^0
  Product : Product  OutDataType=sfix(16)  OutScaling=2^0  RndMeth=Zero
  Sign : Signum  ZeroCross=off
  dF_x/dF_z table : Lookup2D  RowIndex=kappa_bp  ColumnIndex=F_z_bp  Table=dFx_dFz_grid'  LookUpMeth=Interpolation-Use End Values  OutDataType=sfix(16)  OutScaling=2^0
  kappa scale : Gain  Gain=1/kappa_sf  ParameterDataType=sfix(16)  ParameterScaling=2^0  OutDataType=sfix(16)  OutScaling=2^0
  dF_x/dF_z : Outport  OutDataType=sfix(16)  OutScaling=2^0
  wires:
  kappa/1 -> Abs/1, Sign/1
  F_z/1 -> F_z scale/1
  kappa scale/1 -> dF_x/dF_z table/1
  F_z scale/1 -> dF_x/dF_z table/2
  dF_x/dF_z table/1 -> F_x unscale/1
  Abs/1 -> kappa scale/1
  F_x unscale/1 -> Product/2
  Product/1 -> dF_x/dF_z/1
  Sign/1 -> Product/1

== system mech_car_library/Tires/Magic 1/Tire Forces and Moments/Longitudinal Force/Transient slip/Tire force derivative wrt kappa ==
  note: Numerical differentiation of the Magic Formula
  kappa : Inport  OutDataType=sfix(16)  OutScaling=2^0
  F_z : Inport  Port=2  OutDataType=sfix(16)  OutScaling=2^0
  Abs : Abs  ZeroCross=off
  F_x unscale : Gain  Gain=F_x_sf  ParameterDataType=sfix(16)  ParameterScaling=2^0  OutDataType=sfix(16)  OutScaling=2^0
  F_z scale : Gain  Gain=1/F_z_sf  ParameterDataType=sfix(16)  ParameterScaling=2^0  OutDataType=sfix(16)  OutScaling=2^0
  dF_x/dkappa table : Lookup2D  RowIndex=kappa_bp  ColumnIndex=F_z_bp  Table=dFx_dkappa_grid'  LookUpMeth=Interpolation-Use End Values  OutDataType=sfix(16)  OutScaling=2^0
  kappa scale : Gain  Gain=1/kappa_sf  ParameterDataType=sfix(16)  ParameterScaling=2^0  OutDataType=sfix(16)  OutScaling=2^0
  dF_x/dkappa : Outport  OutDataType=sfix(16)  OutScaling=2^0
  wires:
  F_x unscale/1 -> dF_x/dkappa/1
  Abs/1 -> kappa scale/1
  dF_x/dkappa table/1 -> F_x unscale/1
  F_z scale/1 -> dF_x/dkappa table/2
  kappa scale/1 -> dF_x/dkappa table/1
  F_z/1 -> F_z scale/1
  kappa/1 -> Abs/1
